simulink model "cosimulation_lte_dsm"  (R2017b)
settings: Solver=FixedStepDiscrete  StartTime=0.0  StopTime=150e6  RelTol=1e-3
libraries: modelsimlib x1
settings Model: Creator=o_cotte  LastModifiedBy=o_cotte

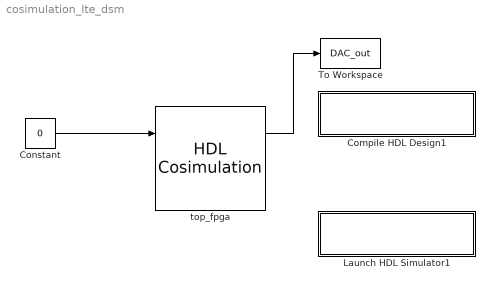
== system cosimulation_lte_dsm ==
  Compile HDL Design1 : Subsystem
      settings: OpenFcn=eval('compile_hdl_design_top_fpga');
      mask Display: disp(['Double-Click to' char(10) 'compile HDL files'])
  Constant : Constant  Value=0  VectorParams1D=off  OutDataTypeStr=boolean
  Launch HDL Simulator1 : Subsystem
      settings: OpenFcn=eval('launch_hdl_simulator_top_fpga');
      mask Display: disp(['Double-Click to' char(10) 'launch HDL simulator'])
  To Workspace : ToWorkspace  VariableName=DAC_out  SampleTime=-1
  top_fpga : modelsimlib/HDL Cosimulation  PortPaths=/top_fpga/bypass;/top_fpga/DAC_in;/top_fpga/DAC_out;/top_fpga/bitstream  PortModes=[1 1 2 2 ]  PortTimes=[-1,-1,1,1]  PortSigns=[-1 -1 1 -1 ]  PortFracLengths=[0,0,32,0]  CommLocal=on  CommSharedMemory=off  CommPortNumber=55990  CommShowInfo=on  ClockModes=[]  ClockTimes=[]  TclPreSimCommand=|  TclPostSimCommand=|  TimingMode=ns  TimingScaleFactor=1  idxCellArray={'UNUSED_VAR'}  CosimBypass=Full Simulation  AllowDirectFeedthrough=on  ProductName=EDA Simulator Link MQ  RunAutoTimescale=off  HdlClocks=/top_fpga/sys_clk 10 ns;  PreRunTime=140  PreRunTimeUnit=ns
      TclPreSimCommand=|
      | force /top_fpga/sys_clk 0 0 ns, 1 5 ns -repeat 10 ns;
      | force /top_fpga/sys_rst 0 0 ns, 1 135 ns;
      TclPostSimCommand=|
      | noforce /top_fpga/sys_clk;
      | noforce /top_fpga/sys_rst;
      | puts "done";
      settings: SourceProductName=HDL Verifier
  wires:
  top_fpga/1 -> To Workspace/1
  Constant/1 -> top_fpga/1

== system cosimulation_lte_dsm/Compile HDL Design1 ==

== system cosimulation_lte_dsm/Launch HDL Simulator1 ==
